simulink model "bt1_ship"  (R2019a)
settings: Solver=ode4  StartTime=0.0  StopTime=4000  FixedStep=0.01  RelTol=1e-3
model workspace (MAT data in the model file):
  k0 = Simulink.Parameter
  k0.DataType = 'auto'
  k0.Dimensions = [0 0]
undefined symbols (not defined in the file): sigbuilder_block
libraries: fuzblock x1
settings Model: Creator=ASUS  LastModifiedBy=ASUS

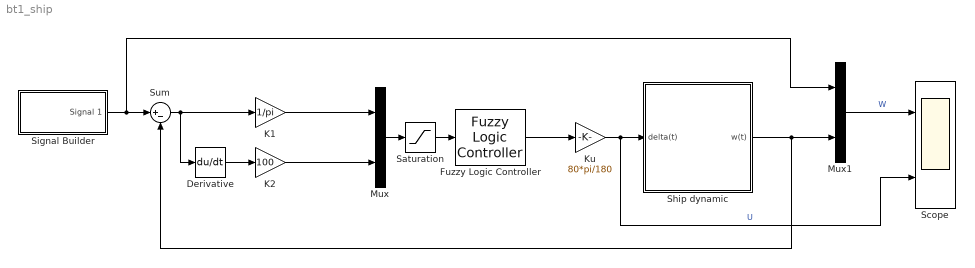
== system bt1_ship ==
  Derivative : Derivative
  Fuzzy Logic Controller : fuzblock/Fuzzy Logic  Controller  FIS='bt1.fis'  OutputSampleNumber=101  DataType=double  FuzzifiedInputs=off  RuleFiringStrengths=off  RuleOutputs=off  AggregatedOutputs=off  SimulateUsing=Interpreted execution  OutOfRangeInputValueMessage=warning  NoRuleFiredMessage=warning  EmptyOutputFuzzySetMessage=warning
  K1 : Gain  Gain=1/pi
  K2 : Gain  Gain=100
  Ku : Gain  Gain=80*pi/180
  Mux : Mux  Inputs=2
  Mux1 : Mux  Inputs=2
  Saturation : Saturate  UpperLimit=1  LowerLimit=-1
  Scope : Scope  NumInputPorts=2
  Ship dynamic : Subsystem  mask{l=161, v=5, k0=-3.86, t10=5.66, t20=0.38, t30=0.89, k=-3.86*5/161, t1=5.66*161/5, t2=0.38*161/5, t3=0.89*161/5}
  Signal Builder : Subsystem  Tag=STV Subsys  LoadFcn=sigbuilder_block('load');  StartFcn=sigbuilder_block('start');  StopFcn=sigbuilder_block('stop');  ClipboardFcn=sigbuilder_block('clipboard');  mask(Sigbuilder block){tuvar=[0:10]}
      mask help: Simulink:masks:SigbuilderBlock_MD
      mask init:
      | if ~strcmp(get_param(bdroot(gcbh),'SimulationStatus'),'stopped') tuvar = sigbuilder_block('maskInit'); end
      settings: CopyFcn=sigbuilder_block('copy');  DeleteFcn=sigbuilder_block('delete');  ModelCloseFcn=sigbuilder_block('modelClose');  PreSaveFcn=sigbuilder_block('preSave');  PauseFcn=sigbuilder_block('pause');  ContinueFcn=sigbuilder_block('continue');  NameChangeFcn=sigbuilder_block('namechange');  OpenFcn=sigbuilder_block('open',[538.8 144.6 550.8 400.2 ]);  CloseFcn=sigbuilder_block('close');
      mask Display: plot(0, 0, 100, 100,[2, 2, 32, 32, 2], [68, 8, 8, 68, 68],[32, 2], [38, 38], [32, 19, 2],[53, 60, 44], [32, 17, 17, 2],[16, 16, 31, 31]);txt = getActiveGroup(gcbh);text(2, 100, txt,'verticalAlignment', 'top');
  Sum : Sum  Inputs=|+-
  wires:
  Ku/1 -> Scope/2, Ship dynamic/1(delta(t))  "U"
  Fuzzy Logic Controller/1 -> Ku/1
  Saturation/1 -> Fuzzy Logic Controller/1
  Mux/1 -> Saturation/1
  Derivative/1 -> K2/1
  Sum/1 -> K1/1, Derivative/1
  K1/1 -> Mux/1
  K2/1 -> Mux/2
  Signal Builder/1(Signal 1) -> Mux1/1, Sum/1
  Ship dynamic/1(w(t)) -> Sum/2, Mux1/2
  Mux1/1 -> Scope/1  "W"

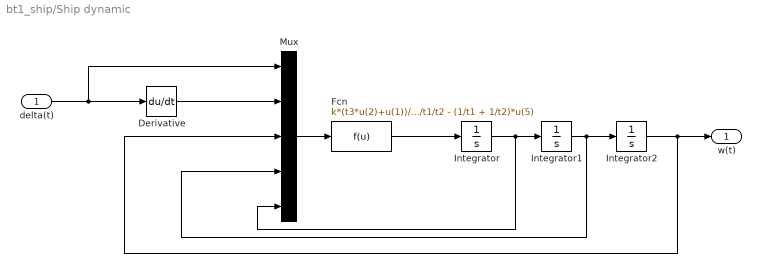
== system bt1_ship/Ship dynamic ==
  delta(t) : Inport
  Derivative : Derivative
  Fcn : Fcn  Expr=k*(t3*u(2)+u(1))/t1/t2 - (u(4)^3+u(4))/t1/t2 - (1/t1 + 1/t2)*u(5)
  Integrator : Integrator
  Integrator1 : Integrator
  Integrator2 : Integrator
  Mux : Mux  Inputs=5
  w(t) : Outport
  wires:
  Fcn/1 -> Integrator/1
  Integrator/1 -> Mux/5, Integrator1/1
  Integrator1/1 -> Mux/4, Integrator2/1
  delta(t)/1 -> Mux/1, Derivative/1
  Derivative/1 -> Mux/2
  Integrator2/1 -> Mux/3, w(t)/1
  Mux/1 -> Fcn/1

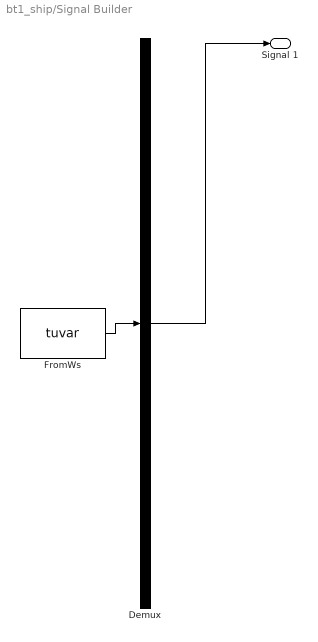
== system bt1_ship/Signal Builder ==
  Demux : Demux  Tag=STV Demux  Outputs=1
  FromWs : FromWorkspace  Tag=STV FromWs  VariableName=tuvar  SampleTime=0
      SigBuilderData=|
      | common.afterFinalStr = 'Extrapolate'
      | common.sampleTime = 0
      | dataSet.timeRange = [0 4000]
      | dataSet.name = 'Group 1'
      | sbobj.Groups.Name = 'Group 1'
      | sbobj.Groups.Signals.Name = 'Signal 1'
      | sbobj.Groups.Signals.XData = [0 1000 1000 2000 2000 3000 3000 4000]
      | sbobj.Groups.Signals.YData = [1.0471975512 1.0471975512 -1.0471975512 -1.0471975512 0.785398163397 0.785398163397 -0.523599 -0.523599]
      | sbobj.Groups.TimeRange = [0 4000]
  Signal 1 : Outport  Tag=STV Outport
  wires:
  Demux/1 -> Signal 1/1
  FromWs/1 -> Demux/1
